simulink model "GearControl"  (R2021b)
settings: Solver=FixedStepDiscrete  StartTime=0.0  StopTime=10.0  FixedStep=1/10  RelTol=1e-3
settings Model: Creator=david  LastModifiedBy=david

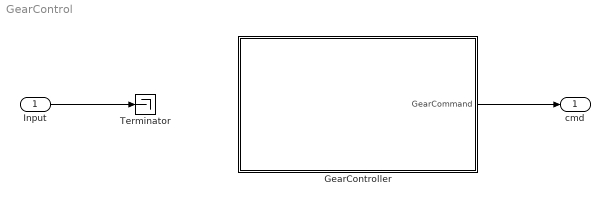
== system GearControl ==
  Input : Inport
  GearController : Stateflow chart  TreatAsAtomicUnit=on
  Terminator : Terminator
  cmd : Outport
  wires:
  GearController/1(GearCommand) -> cmd/1
  Input/1 -> Terminator/1

== stateflow chart GearControl/GearController ==
  state EntryState
    entry:
    GearCommand = GearPosition.down;
  state GearUp
  state GearDown
  (default) -> EntryState
  EntryState -> GearDown [order 1] : [GearCommand == GearPosition.down]
  EntryState -> GearUp [order 2] : [GearCommand == GearPosition.up]
  data: GearCommand output =GearPosition.down
